simulink model "Simulink"  (R2022b)
settings: Solver=ode4  StartTime=0.0  StopTime=0.04  FixedStep=0.000010  RelTol=1e-3
values from neighbouring files (symbols this model uses):
  CFreq = 1080    [main.mat]    (also in main1.m)
  Lload = 0.01    [main.mat]    (also in main1.m)
  Rload = 2    [main.mat]    (also in main1.m)
  Vdc = 250    [main.mat]    (also in main1.m)
libraries: simulink x1, spspowerguiLib x1
settings Model: Creator=pouyaalaei  LastModifiedBy=igho
settings SolverCC: AlgebraicLoopSolver=TrustRegion
settings DataIOCC: ReturnWorkspaceOutputs=off
settings DebuggingCC: UnconnectedInputMsg=warning  UnconnectedOutputMsg=warning  UnconnectedLineMsg=warning  SFMachineParentedDataDiag=warning
settings ModelReferenceCC: EnableRefExpFcnMdlSchedulingChecks=on
settings RTWCC: DLArmComputeVersion=19.05

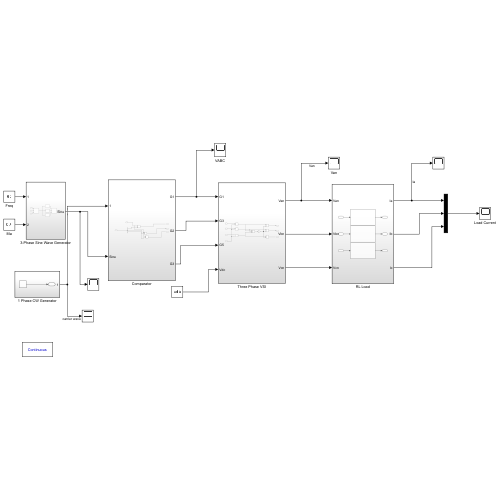
[thumbnail: Simulink's stored preview of the top-level diagram]
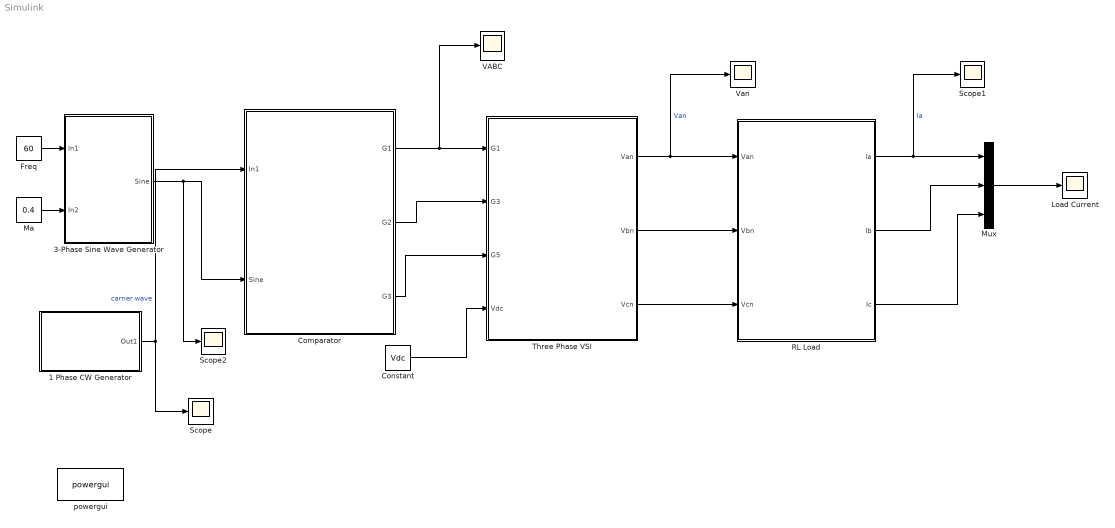
== system Simulink ==
  1 Phase CW Generator : Subsystem
  3-Phase Sine Wave Generator : Subsystem
  Comparator : Subsystem
  Constant : Constant  Value=Vdc
  Freq : Constant  Value=60
  Load Current : Scope
  Ma : Constant  Value=0.4
  Mux : Mux  Inputs=3
  RL Load : Subsystem
  Scope : Scope
  Scope1 : Scope
  Scope2 : Scope
  Three Phase VSI : Subsystem
  VABC : Scope
  Van : Scope
  powergui : spspowerguiLib/powergui  Priority=1  SimulationMode=Continuous  SampleTime=50e-6  frequency=60  Iterations=50  frequencyindice=60  Pbase=100e6  ErrMax=1e-4  UnitsV=kV  UnitsW=MW  buscounter=0  FunctionMessages=off  echomessages=off  EnableUseOfTLC=off  CurrentSourceSwitches=off  DisableSnubberDevices=off  DisableRonSwitches=off  DisableVfSwitches=off  DisplayEquations=off  AutomaticDiscreteSolvers=off  SolverType=Tustin/Backward Euler (TBE)  Interpol=off  ExternalGateDelay=off  methode=off  Ts=100  x0status=blocks  SPID=on  SwTol=0  HookPort=off  NonlinearTolerance=1e-4  nMaxIteration=100  ContinueOnMaxIteration=off  RestoreLinks=warning  ResistiveCurrentMeasurement=off  Frange=[0:2:500]  Ylog=off  Xlog=on  ShowGrid=off  save=off  variable=ZData  structure=0  ZoomFFT=off  StartTime=0.0  cycles=1  DisplayStyle=1  fundamental=60  FreqAxis=off  MaxFrequency=1000  frequencyindicesteady=1  RmsSteady=1  display=off
  wires:
  Constant/1 -> Three Phase VSI/4(Vdc)
  Three Phase VSI/1(Van) -> Van/1, RL Load/1(Van)  "Van"
  Three Phase VSI/2(Vbn) -> RL Load/2(Vbn)
  Three Phase VSI/3(Vcn) -> RL Load/3(Vcn)
  RL Load/1(Ia) -> Scope1/1, Mux/1  "Ia"
  RL Load/2(Ib) -> Mux/2
  RL Load/3(Ic) -> Mux/3
  Mux/1 -> Load Current/1
  Ma/1 -> 3-Phase Sine Wave Generator/2(In2)
  Freq/1 -> 3-Phase Sine Wave Generator/1(In1)
  1 Phase CW Generator/1(Out1) -> Scope/1, Comparator/1(In1)  "carrier wave"
  3-Phase Sine Wave Generator/1(Sine) -> Scope2/1, Comparator/2(Sine)
  Comparator/1(G1) -> VABC/1, Three Phase VSI/1(G1)
  Comparator/2(G2) -> Three Phase VSI/2(G3)
  Comparator/3(G3) -> Three Phase VSI/3(G5)

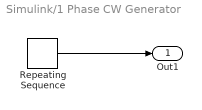
== system Simulink/1 Phase CW Generator ==
  Repeating Sequence : simulink/Sources/Repeating Sequence  rep_seq_t=[0 1/CFreq/4 3/CFreq/4 1/CFreq]  rep_seq_y=[0 1 -1 0]
  Out1 : Outport
  wires:
  Repeating Sequence/1 -> Out1/1

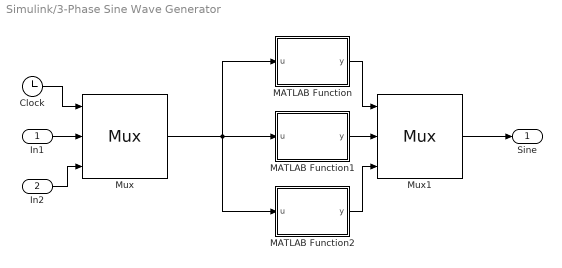
== system Simulink/3-Phase Sine Wave Generator ==
  In1 : Inport
  In2 : Inport  Port=2
  Clock : Clock
  MATLAB Function : MATLAB Function  TreatAsAtomicUnit=on
  MATLAB Function1 : MATLAB Function  TreatAsAtomicUnit=on
  MATLAB Function2 : MATLAB Function  TreatAsAtomicUnit=on
  Mux : Mux  Inputs=3
  Mux1 : Mux  Inputs=3
  Sine : Outport
  wires:
  Clock/1 -> Mux/1
  In1/1 -> Mux/2
  In2/1 -> Mux/3
  Mux/1 -> MATLAB Function/1(u), MATLAB Function2/1(u), MATLAB Function1/1(u)
  Mux1/1 -> Sine/1
  MATLAB Function/1(y) -> Mux1/1
  MATLAB Function2/1(y) -> Mux1/3
  MATLAB Function1/1(y) -> Mux1/2

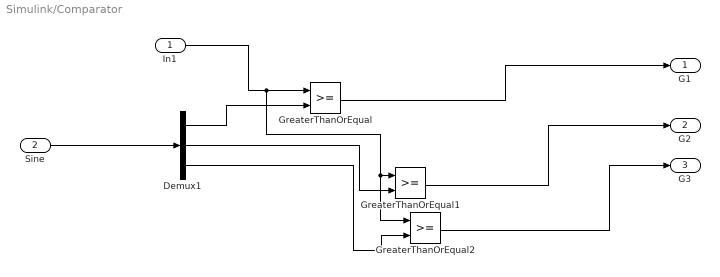
== system Simulink/Comparator ==
  In1 : Inport
  Sine : Inport  Port=2
  Demux1 : Demux  Outputs=3
  GreaterThanOrEqual : RelationalOperator  OutDataTypeStr=boolean  RndMeth=Simplest  InputSameDT=off
  GreaterThanOrEqual1 : RelationalOperator  OutDataTypeStr=boolean  RndMeth=Simplest  InputSameDT=off
  GreaterThanOrEqual2 : RelationalOperator  OutDataTypeStr=boolean  RndMeth=Simplest  InputSameDT=off
  G1 : Outport
  G2 : Outport  Port=2
  G3 : Outport  Port=3
  wires:
  In1/1 -> GreaterThanOrEqual1/1, GreaterThanOrEqual2/1, GreaterThanOrEqual/1
  Sine/1 -> Demux1/1
  GreaterThanOrEqual1/1 -> G2/1
  GreaterThanOrEqual2/1 -> G3/1
  Demux1/2 -> GreaterThanOrEqual1/2
  Demux1/1 -> GreaterThanOrEqual/2
  Demux1/3 -> GreaterThanOrEqual2/2
  GreaterThanOrEqual/1 -> G1/1

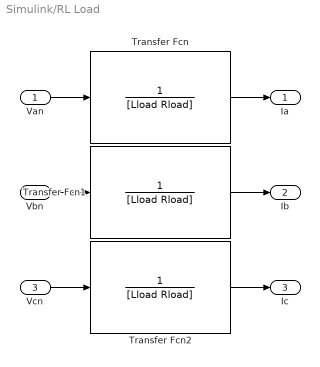
== system Simulink/RL Load ==
  Van : Inport
  Vbn : Inport  Port=2
  Vcn : Inport  Port=3
  Transfer Fcn : TransferFcn  Denominator=[Lload Rload]
  Transfer Fcn1 : TransferFcn  Denominator=[Lload Rload]
  Transfer Fcn2 : TransferFcn  Denominator=[Lload Rload]
  Ia : Outport
  Ib : Outport  Port=2
  Ic : Outport  Port=3
  wires:
  Van/1 -> Transfer Fcn/1
  Vbn/1 -> Transfer Fcn1/1
  Vcn/1 -> Transfer Fcn2/1
  Transfer Fcn2/1 -> Ic/1
  Transfer Fcn1/1 -> Ib/1
  Transfer Fcn/1 -> Ia/1

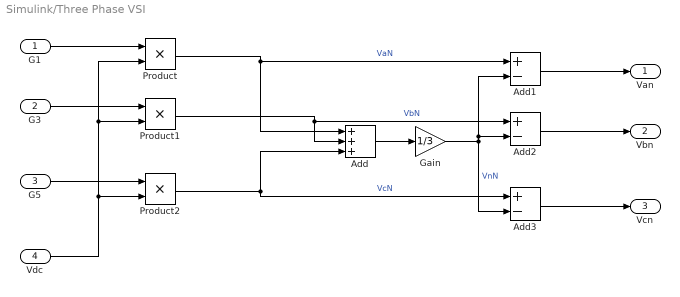
== system Simulink/Three Phase VSI ==
  G1 : Inport
  G3 : Inport  Port=2
  G5 : Inport  Port=3
  Vdc : Inport  Port=4
  Add : Sum  Inputs=+++
  Add1 : Sum  Inputs=+-
  Add2 : Sum  Inputs=+-
  Add3 : Sum  Inputs=+-
  Gain : Gain  Gain=1/3
  Product : Product
  Product1 : Product
  Product2 : Product
  Van : Outport
  Vbn : Outport  Port=2
  Vcn : Outport  Port=3
  wires:
  G3/1 -> Product1/1
  G1/1 -> Product/1
  G5/1 -> Product2/1
  Vdc/1 -> Product/2, Product1/2, Product2/2
  Product/1 -> Add1/1, Add/1  "VaN"
  Product1/1 -> Add2/1, Add/2  "VbN"
  Product2/1 -> Add/3, Add3/1  "VcN"
  Add/1 -> Gain/1
  Gain/1 -> Add1/2, Add2/2, Add3/2  "VnN"
  Add1/1 -> Van/1
  Add2/1 -> Vbn/1
  Add3/1 -> Vcn/1

== matlab function Simulink/3-Phase Sine Wave Generator/MATLAB Function ==
  data: u input; y output
function y = fcn(u)


y = u(3)*sin(2*pi*u(2)*u(1));

== matlab function Simulink/3-Phase Sine Wave Generator/MATLAB Function2 ==
  data: u input; y output
function y = fcn(u)

y = u(3)*sin(2*pi*u(2)*u(1)+(2*pi/3));

== matlab function Simulink/3-Phase Sine Wave Generator/MATLAB Function1 ==
  data: u input; y output
function y = fcn(u)

y = u(3)*sin(2*pi*u(2)*u(1)-(2*pi/3));
